simulink model "figure_5_Air_control_block"  (R2021a)
settings: Solver=VariableStepAuto  StartTime=0.0  StopTime=10.0  RelTol=1e-3
model workspace (MAT data in the model file):
  Tw = Simulink.Parameter
  Tw.DataType = 'auto'
  Tw.Dimensions = [0 0]
settings Model: Creator=user  LastModifiedBy=user

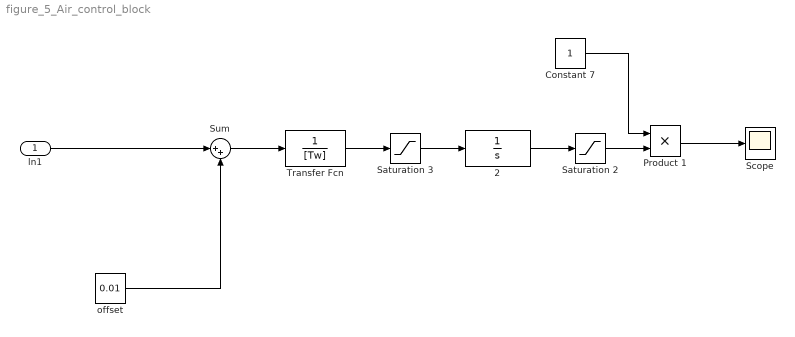
== system figure_5_Air_control_block ==
  ln1 : Inport
  2 : TransferFcn  Denominator=[1 0]
  Constant 7 : Constant
  Product 1 : Product
  Saturation 2 : Saturate
  Saturation 3 : Saturate
  Scope : Scope
  Sum : Sum  Inputs=|++
  Transfer Fcn : TransferFcn  Denominator=[Tw]
  offset : Constant  Value=0.01
  wires:
  ln1/1 -> Sum/1
  offset/1 -> Sum/2
  Sum/1 -> Transfer Fcn/1
  Transfer Fcn/1 -> Saturation 3/1
  Saturation 3/1 -> 2/1
  2/1 -> Saturation 2/1
  Saturation 2/1 -> Product 1/2
  Constant 7/1 -> Product 1/1
  Product 1/1 -> Scope/1
